simulink model "controller"  (R2022b)
settings: Solver=FixedStepAuto  StartTime=0.0  StopTime=10.0  FixedStep=0.01  RelTol=1e-3
undefined symbols (not defined in the file): MI_STATUSES
libraries: battery_monitor_lib x1, driver_interface_lib x1, governor_lib x1, motor_interface_lib x1, vehicle_dynamics_lib x1
settings Model: Creator=dr_pa  LastModifiedBy=LinF
settings DataIOCC: ExternalInput=Testbench_startup.getElement('AMK_bReserve'),Testbench_startup.getElement('DI_V_SteeringAngle'),Testbench_startup.getElement('DI_V_BrakePedalPos'),Testbench_startup.getElement('DI_b_DriverButton'),Testbench_startup.getElement('DI_V_AccelPedalPos1'),Testbench_startup.getElement('DI_V_AccelPedalPos2'),Testbench_startup.getElement('BM_b_prechrgContactorSts'),Testbench_startup.getElement('BM_b_HVposContactorSts'),Testbench_startup.getElement('BM_b_HVnegContactorSts'),Testbench_startup.getElement('AMK_bSystemReady'),Testbench_startup.getElement('AMK_bError'),Testbench_startup.getElement('AMK_bWarn'),Testbench_startup.getElement('AMK_bQuitDcOn'),Testbench_startup.getElement('AMK_bDcOn'),Testbench_startup.getElement('AMK_bQuitInverterOn'),Testbench_startup.getElement('AMK_bInverterOn'),Testbench_startup.getElement('AMK_bDerating'),Testbench_startup.getElement('AMK_TempMotor'),Testbench_startup.getElement('AMK_TempInverter'),Testbench_startup.getElement('AMK_ErrorInfo'),Testbench_startup.getElement('AMK_TempIGBT'),Testbench_startup.getElement('AMK_ActualVelocity'),Testbench_startup.getElement('AMK_TorqueCurrent'),Testbench_startup.getElement('AMK_MagnetizingCurrent')  LoadExternalInput=on
settings OptimizationCC: DefaultParameterBehavior=Inlined  EnhancedBackFolding=on  PassReuseOutputArgsAs=Individual arguments  ZeroExternalMemoryAtStartup=off  ZeroInternalMemoryAtStartup=off  OptimizeBlockOrder=speed  DifferentSizesBufferReuse=on  OptimizationCustomize=off  EfficientTunableParamExpr=on
settings DebuggingCC: ParameterTunabilityLossMsg=error
settings SFSimCC: MATLABDynamicMemAlloc=off
settings RTWCC: Description=Embedded Coder  SystemTargetFile=ert.tlc  GenCodeOnly=on  TemplateMakefile=ert_default_tmf
settings CodeAppCC: ForceParamTrailComments=on  IgnoreCustomStorageClasses=off  OperatorAnnotations=on  SimulinkDataObjDesc=on  SFDataObjDesc=on  InsertBlockDesc=on
settings ERTTargetCC: TargetLangStandard=C99 (ISO)  GenerateSampleERTMain=on  InlinedParameterPlacement=NonHierarchical  ERTCustomFileTemplate=example_file_process.tlc

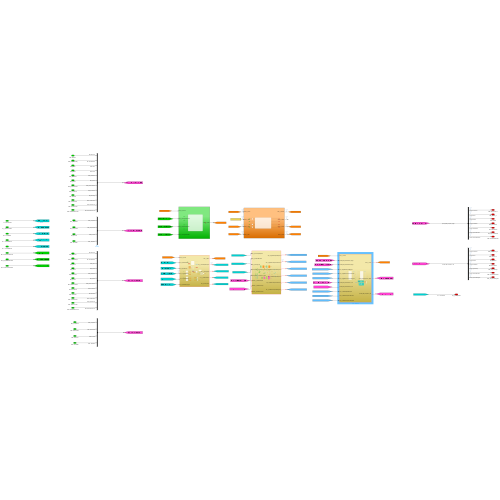
[thumbnail: Simulink's stored preview of the top-level diagram]
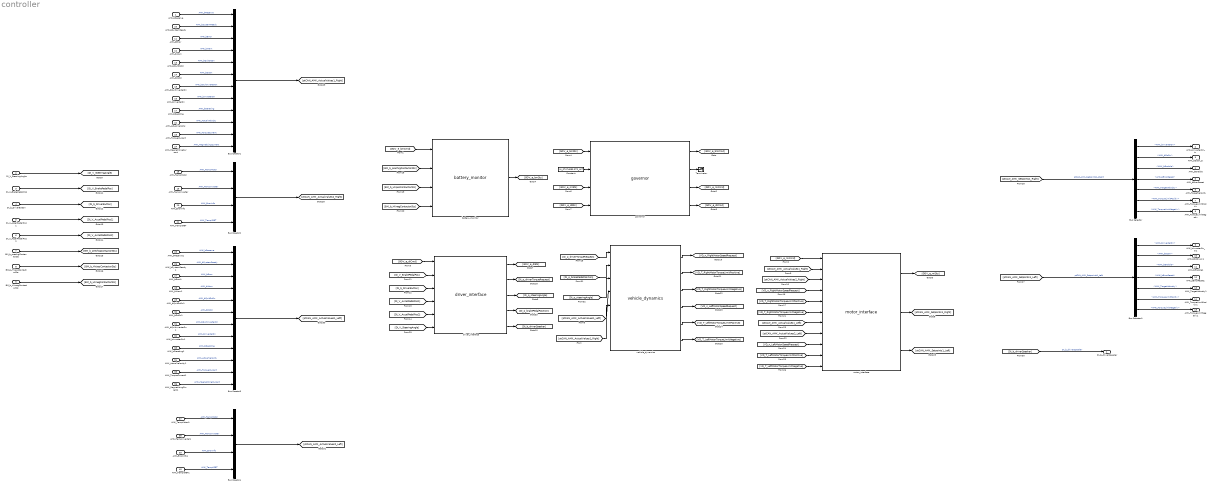
== system controller ==
  AMK_bReserve : Inport  OutDataTypeStr=boolean  Unit=uint64
  DI_V_SteeringAngle : Inport  Port=2  OutDataTypeStr=int16
  DI_V_BrakePedalPos : Inport  Port=3  OutDataTypeStr=int16
  DI_b_DriverButton : Inport  Port=4  OutDataTypeStr=boolean
  DI_V_AccelPedalPos1 : Inport  Port=5  OutDataTypeStr=int16
  DI_V_AccelPedalPos2 : Inport  Port=6  OutDataTypeStr=int16
  BM_b_prechrgContactorSts : Inport  Port=7  OutDataTypeStr=boolean
  BM_b_HVposContactorSts : Inport  Port=8  OutDataTypeStr=boolean
  BM_b_HVnegContactorSts : Inport  Port=9  OutDataTypeStr=boolean
  AMK_bSystemReady : Inport  Port=10  OutDataTypeStr=boolean  Unit=uint64
  AMK_bError : Inport  Port=11  OutDataTypeStr=boolean  Unit=uint64
  AMK_bWarn : Inport  Port=12  OutDataTypeStr=boolean  Unit=uint64
  AMK_bQuitDcOn : Inport  Port=13  OutDataTypeStr=boolean  Unit=uint64
  AMK_bDcOn : Inport  Port=14  OutDataTypeStr=boolean  Unit=uint64
  AMK_bQuitInverterOn : Inport  Port=15  OutDataTypeStr=boolean  Unit=uint64
  AMK_bInverterOn : Inport  Port=16  OutDataTypeStr=boolean  Unit=uint64
  AMK_bDerating : Inport  Port=17  OutDataTypeStr=boolean  Unit=uint64
  AMK_TempMotor : Inport  Port=18  OutDataTypeStr=int16  Unit=uint64
  AMK_TempInverter : Inport  Port=19  OutDataTypeStr=int16  Unit=uint64
  AMK_ErrorInfo : Inport  Port=20  OutDataTypeStr=uint16
  AMK_TempIGBT : Inport  Port=21  OutDataTypeStr=int16
  AMK_ActualVelocity : Inport  Port=22  OutDataTypeStr=int16  Unit=uint64
  AMK_TorqueCurrent : Inport  Port=23  OutDataTypeStr=int16  Unit=uint64
  AMK_MagnetizingCurrent : Inport  Port=24  OutDataTypeStr=int16  Unit=uint64
  AMK_bReserve1 : Inport  Port=25  OutDataTypeStr=boolean  Unit=uint64
  AMK_bSystemReady1 : Inport  Port=26  OutDataTypeStr=boolean  Unit=uint64
  AMK_bError1 : Inport  Port=27  OutDataTypeStr=boolean  Unit=uint64
  AMK_bWarn1 : Inport  Port=28  OutDataTypeStr=boolean  Unit=uint64
  AMK_bQuitDcOn1 : Inport  Port=29  OutDataTypeStr=boolean  Unit=uint64
  AMK_bDcOn1 : Inport  Port=30  OutDataTypeStr=boolean  Unit=uint64
  AMK_bQuitInverterOn1 : Inport  Port=31  OutDataTypeStr=boolean  Unit=uint64
  AMK_bInverterOn1 : Inport  Port=32  OutDataTypeStr=boolean  Unit=uint64
  AMK_bDerating1 : Inport  Port=33  OutDataTypeStr=boolean  Unit=uint64
  AMK_ActualVelocity1 : Inport  Port=34  OutDataTypeStr=int16  Unit=uint64
  AMK_TorqueCurrent1 : Inport  Port=35  OutDataTypeStr=int16  Unit=uint64
  AMK_MagnetizingCurrent1 : Inport  Port=36  OutDataTypeStr=int16  Unit=uint64
  AMK_TempMotor1 : Inport  Port=37  OutDataTypeStr=int16  Unit=uint64
  AMK_TempInverter1 : Inport  Port=38  OutDataTypeStr=int16  Unit=uint64
  AMK_ErrorInfo1 : Inport  Port=39  OutDataTypeStr=uint16
  AMK_TempIGBT1 : Inport  Port=40  OutDataTypeStr=int16
  Bus Creator1 : BusCreator  Inputs=12
  Bus Creator2 : BusCreator  Inputs=4
  Bus Creator3 : BusCreator  Inputs=12
  Bus Creator4 : BusCreator  Inputs=4
  Bus Selector : BusSelector  OutputSignals=AMK_bInverterOn,AMK_bDcOn,AMK_bEnable,AMK_bErrorReset,AMK_TargetVelocity,AMK_TorqueLimitPositiv,AMK_TorqueLimitNegativ
  Bus Selector1 : BusSelector  OutputSignals=AMK_bInverterOn,AMK_bDcOn,AMK_bEnable,AMK_bErrorReset,AMK_TargetVelocity,AMK_TorqueLimitPositiv,AMK_TorqueLimitNegativ
  Constant : Constant  Value=MI_STATUSES.STS_INIT  OutDataTypeStr=Enum: MI_STATUSES
  Terminator : Terminator
  battery_monitor : battery_monitor_lib/battery_monitor  SystemSampleTime=-1  VariantActivationTime=update diagram  Latency=0  AutoFrameSizeCalculation=off
  driver_interface : driver_interface_lib/driver_interface  SystemSampleTime=-1  VariantActivationTime=update diagram  Latency=0  AutoFrameSizeCalculation=off
  governor : governor_lib/governor  SystemSampleTime=-1  VariantActivationTime=update diagram  Latency=0  AutoFrameSizeCalculation=off
  motor_interface : motor_interface_lib/motor_interface  SystemSampleTime=-1  VariantActivationTime=update diagram  Latency=0  AutoFrameSizeCalculation=off
  vehicle_dynamics : vehicle_dynamics_lib/vehicle_dynamics  SystemSampleTime=-1  VariantActivationTime=update diagram  Latency=0  AutoFrameSizeCalculation=off
  DI_b_driverSpeaker : Outport
  AMK_bInverterOn_tx : Outport  Port=2
  AMK_bDcOn_tx : Outport  Port=3
  AMK_bEnable : Outport  Port=4
  AMK_bErrorReset : Outport  Port=5
  AMK_TargetVelocity : Outport  Port=6
  AMK_TorqueLimitPositiv : Outport  Port=7
  AMK_TorqueLimitNegativ : Outport  Port=8
  AMK_bInverterOn_tx1 : Outport  Port=9
  AMK_bDcOn_tx1 : Outport  Port=10
  AMK_bEnable1 : Outport  Port=11
  AMK_bErrorReset1 : Outport  Port=12
  AMK_TargetVelocity1 : Outport  Port=13
  AMK_TorqueLimitPositiv1 : Outport  Port=14
  AMK_TorqueLimitNegativ1 : Outport  Port=15
  wires:
  driver_interface/3 -> [DI_p_steeringAngle]
  driver_interface/5 -> [DI_b_driverSpeaker]
  [GOV_e_miSts] -> governor/3
  [BM_b_HVposContactorSts] -> battery_monitor/3
  vehicle_dynamics/6 -> [VD_T_LeftMotorTorqueLimitNegative]
  vehicle_dynamics/4 -> [VD_n_LeftMotorSpeedRequest]
  [VD_T_RightMotorTorqueLimitPositive] -> motor_interface/5
  driver_interface/4 -> [DI_p_brakePedalPosition]
  [GOV_e_diCmd] -> driver_interface/1
  BM_b_HVnegContactorSts/1 -> [BM_b_HVnegContactorSts]
  [ptCAN_AMK_Setpoints1_Left] -> Bus Selector1/1  "ptCAN_AMK_Setpoints1_Left"
  [DI_p_steeringAngle] -> vehicle_dynamics/3
  vehicle_dynamics/3 -> [VD_T_RightMotorTorqueLimitNegative]
  vehicle_dynamics/1 -> [VD_n_RightMotorSpeedRequest]
  [DI_b_driverSpeaker] -> DI_b_driverSpeaker/1  "DI_b_driverSpeaker"
  [ptCAN_AMK_ActualValues1_Left] -> vehicle_dynamics/4
  [VD_T_RightMotorTorqueLimitNegative] -> motor_interface/6
  [ptCAN_AMK_ActualValues1_Right] -> vehicle_dynamics/5
  [DI_p_driverTorqueRequest] -> vehicle_dynamics/1
  [DI_V_SteeringAngle] -> driver_interface/6
  [GOV_e_bmCmd] -> battery_monitor/1
  [BM_b_HVnegContactorSts] -> battery_monitor/4
  vehicle_dynamics/2 -> [VD_T_RightMotorTorqueLimitPositive]
  driver_interface/2 -> [DI_p_driverTorqueRequest]
  [DI_b_DriverButton] -> driver_interface/3
  [DI_V_AccelPedalPos1] -> driver_interface/4
  DI_V_BrakePedalPos/1 -> [DI_V_BrakePedalPos]
  [BM_b_prechrgContactorSts] -> battery_monitor/2
  [DI_V_AccelPedalPos2] -> driver_interface/5
  driver_interface/1 -> [GOV_e_diSts]
  Constant/1 -> governor/2
  [ptCAN_AMK_ActualValues2_Right] -> motor_interface/3
  [GOV_e_bmSts] -> governor/1
  battery_monitor/1 -> [GOV_e_bmSts]
  [VD_n_RightMotorSpeedRequest] -> motor_interface/4
  DI_V_AccelPedalPos2/1 -> [DI_V_AccelPedalPos2]
  vehicle_dynamics/5 -> [VD_T_LeftMotorTorqueLimitPositive]
  governor/3 -> [GOV_e_miCmd]
  [GOV_e_diSts] -> governor/4
  [ptCAN_AMK_Setpoints1_Right] -> Bus Selector/1  "ptCAN_AMK_Setpoints1_Right"
  [DI_V_BrakePedalPos] -> driver_interface/2
  DI_b_DriverButton/1 -> [DI_b_DriverButton]
  BM_b_prechrgContactorSts/1 -> [BM_b_prechrgContactorSts]
  [GOV_e_miCmd] -> motor_interface/1
  governor/4 -> [GOV_e_diCmd]
  [ptCAN_AMK_ActualValues1_Right] -> motor_interface/2
  DI_V_AccelPedalPos1/1 -> [DI_V_AccelPedalPos1]
  governor/2 -> Terminator/1
  motor_interface/1 -> [GOV_e_miSts]
  BM_b_HVposContactorSts/1 -> [BM_b_HVposContactorSts]
  [DI_p_brakePedalPosition] -> vehicle_dynamics/2
  governor/1 -> [GOV_e_bmCmd]
  motor_interface/2 -> [ptCAN_AMK_Setpoints1_Right]
  DI_V_SteeringAngle/1 -> [DI_V_SteeringAngle]
  AMK_bSystemReady/1 -> Bus Creator1/2  "AMK_bSystemReady"
  AMK_bDerating/1 -> Bus Creator1/9  "AMK_bDerating"
  Bus Creator1/1 -> [ptCAN_AMK_ActualValues1_Right]
  AMK_bQuitDcOn/1 -> Bus Creator1/5  "AMK_bQuitDcOn"
  AMK_bQuitInverterOn/1 -> Bus Creator1/7  "AMK_bQuitInverterOn"
  AMK_TempInverter/1 -> Bus Creator2/2  "AMK_TempInverter"
  AMK_bDcOn/1 -> Bus Creator1/6  "AMK_bDcOn"
  AMK_bReserve/1 -> Bus Creator1/1  "AMK_bReserve"
  AMK_bWarn/1 -> Bus Creator1/4  "AMK_bWarn"
  AMK_ActualVelocity/1 -> Bus Creator1/10  "AMK_ActualVelocity"
  AMK_bError/1 -> Bus Creator1/3  "AMK_bError"
  AMK_TempMotor/1 -> Bus Creator2/1  "AMK_TempMotor"
  AMK_TorqueCurrent/1 -> Bus Creator1/11  "AMK_TorqueCurrent"
  AMK_TempIGBT/1 -> Bus Creator2/4  "AMK_TempIGBT"
  AMK_ErrorInfo/1 -> Bus Creator2/3  "AMK_ErrorInfo"
  AMK_MagnetizingCurrent/1 -> Bus Creator1/12  "AMK_MagnetizingCurrent"
  Bus Creator2/1 -> [ptCAN_AMK_ActualValues2_Right]
  AMK_bInverterOn/1 -> Bus Creator1/8  "AMK_bInverterOn"
  motor_interface/3 -> [ptCAN_AMK_Setpoints1_Left]
  [ptCAN_AMK_ActualValues1_Left] -> motor_interface/7
  [ptCAN_AMK_ActualValues2_Left] -> motor_interface/8
  [VD_n_LeftMotorSpeedRequest] -> motor_interface/9
  [VD_T_LeftMotorTorqueLimitPositive] -> motor_interface/10
  [VD_T_LeftMotorTorqueLimitNegative] -> motor_interface/11
  Bus Selector/4 -> AMK_bErrorReset/1  "<AMK_bErrorReset>"
  Bus Selector/5 -> AMK_TargetVelocity/1  "<AMK_TargetVelocity>"
  Bus Selector/1 -> AMK_bInverterOn_tx/1  "<AMK_bInverterOn>"
  Bus Selector/2 -> AMK_bDcOn_tx/1  "<AMK_bDcOn>"
  Bus Selector/6 -> AMK_TorqueLimitPositiv/1  "<AMK_TorqueLimitPositiv>"
  Bus Selector/3 -> AMK_bEnable/1  "<AMK_bEnable>"
  Bus Selector/7 -> AMK_TorqueLimitNegativ/1  "<AMK_TorqueLimitNegativ>"
  Bus Selector1/3 -> AMK_bEnable1/1  "<AMK_bEnable>"
  Bus Selector1/2 -> AMK_bDcOn_tx1/1  "<AMK_bDcOn>"
  Bus Selector1/5 -> AMK_TargetVelocity1/1  "<AMK_TargetVelocity>"
  Bus Selector1/1 -> AMK_bInverterOn_tx1/1  "<AMK_bInverterOn>"
  Bus Selector1/4 -> AMK_bErrorReset1/1  "<AMK_bErrorReset>"
  Bus Selector1/6 -> AMK_TorqueLimitPositiv1/1  "<AMK_TorqueLimitPositiv>"
  Bus Selector1/7 -> AMK_TorqueLimitNegativ1/1  "<AMK_TorqueLimitNegativ>"
  AMK_MagnetizingCurrent1/1 -> Bus Creator3/12  "AMK_MagnetizingCurrent"
  Bus Creator3/1 -> [ptCAN_AMK_ActualValues1_Left]
  AMK_bInverterOn1/1 -> Bus Creator3/8  "AMK_bInverterOn"
  AMK_bError1/1 -> Bus Creator3/3  "AMK_bError"
  AMK_bWarn1/1 -> Bus Creator3/4  "AMK_bWarn"
  AMK_ActualVelocity1/1 -> Bus Creator3/10  "AMK_ActualVelocity"
  AMK_TorqueCurrent1/1 -> Bus Creator3/11  "AMK_TorqueCurrent"
  AMK_bQuitInverterOn1/1 -> Bus Creator3/7  "AMK_bQuitInverterOn"
  AMK_bDcOn1/1 -> Bus Creator3/6  "AMK_bDcOn"
  AMK_bQuitDcOn1/1 -> Bus Creator3/5  "AMK_bQuitDcOn"
  AMK_bDerating1/1 -> Bus Creator3/9  "AMK_bDerating"
  AMK_bReserve1/1 -> Bus Creator3/1  "AMK_bReserve"
  AMK_bSystemReady1/1 -> Bus Creator3/2  "AMK_bSystemReady"
  AMK_TempInverter1/1 -> Bus Creator4/2  "AMK_TempInverter"
  AMK_TempIGBT1/1 -> Bus Creator4/4  "AMK_TempIGBT"
  AMK_ErrorInfo1/1 -> Bus Creator4/3  "AMK_ErrorInfo"
  Bus Creator4/1 -> [ptCAN_AMK_ActualValues2_Left]
  AMK_TempMotor1/1 -> Bus Creator4/1  "AMK_TempMotor"
